simulink model "Buck_BLDC_2023a_4_FaultModel"  (R2024a)
settings: Solver=VariableStepAuto  StartTime=0.0  StopTime=35  RelTol=1e-3  EnableMultiTasking=on
model workspace (MAT data in the model file):
  encoderResolution = 2000
  hallOffset = '0.5'
  indexOffset = 850
  polePairs = '4'
settings Model: Creator=feder  LastModifiedBy=feder
settings OptimizationCC: DefaultParameterBehavior=Inlined
settings DebuggingCC: InheritedTsInSrcMsg=none

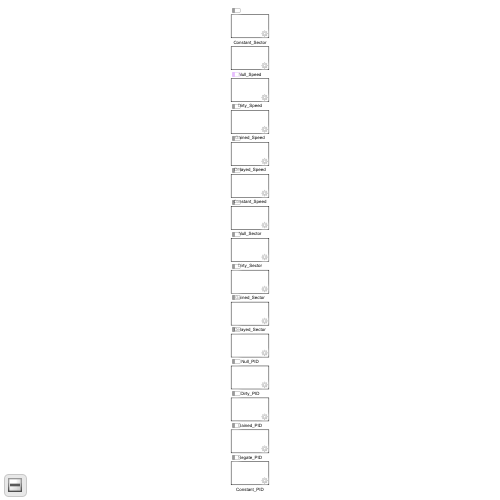
[thumbnail: Simulink's stored preview of the top-level diagram]
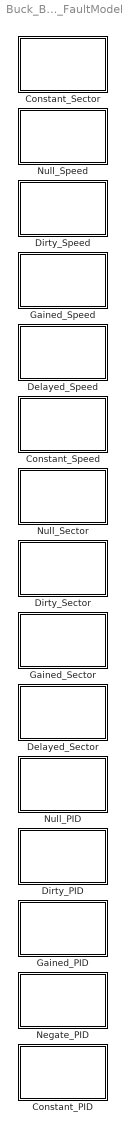
== system Buck_BLDC_2023a_4_FaultModel ==
  Constant_PID : Subsystem  TreatAsAtomicUnit=on  ScheduleAs=Aperiodic partition  PartitionName=PartitionFor_Constant_PID_4698_000977  IsInjectorSS=on
      settings: LibrarySourceBlock=mwfaultlib/Stuck-at-Constant
  Constant_Sector : Subsystem  TreatAsAtomicUnit=on  ScheduleAs=Aperiodic partition  PartitionName=PartitionFor_Constant_Sector_1447_001221  IsInjectorSS=on
      settings: LibrarySourceBlock=mwfaultlib/Stuck-at-Constant
  Constant_Speed : Subsystem  TreatAsAtomicUnit=on  ScheduleAs=Aperiodic partition  PartitionName=PartitionFor_Constant_Speed_1366_012451  IsInjectorSS=on
      settings: LibrarySourceBlock=mwfaultlib/Stuck-at-Constant
  Delayed_Sector : Subsystem  TreatAsAtomicUnit=on  ScheduleAs=Aperiodic partition  PartitionName=PartitionFor_Delayed_Sector_4477_001099  IsInjectorSS=on
      settings: LibrarySourceBlock=mwfaultlib/Unit Delay
  Delayed_Speed : Subsystem  TreatAsAtomicUnit=on  ScheduleAs=Aperiodic partition  PartitionName=PartitionFor_Delayed_Speed_4718_000854  IsInjectorSS=on
      settings: LibrarySourceBlock=mwfaultlib/Unit Delay
  Dirty_PID : Subsystem  TreatAsAtomicUnit=on  ScheduleAs=Aperiodic partition  PartitionName=PartitionFor_Dirty_PID_4657_000854  IsInjectorSS=on
      settings: LibrarySourceBlock=mwfaultlib/Add Noise
  Dirty_Sector : Subsystem  TreatAsAtomicUnit=on  ScheduleAs=Aperiodic partition  PartitionName=PartitionFor_Dirty_Sector_4453_001221  IsInjectorSS=on
      settings: LibrarySourceBlock=mwfaultlib/Add Noise
  Dirty_Speed : Subsystem  TreatAsAtomicUnit=on  ScheduleAs=Aperiodic partition  PartitionName=PartitionFor_Dirty_Speed_7587_001343  IsInjectorSS=on
      settings: LibrarySourceBlock=mwfaultlib/Add Noise
  Gained_PID : Subsystem  TreatAsAtomicUnit=on  ScheduleAs=Aperiodic partition  PartitionName=PartitionFor_Gained_PID_4671_001221  IsInjectorSS=on
      settings: LibrarySourceBlock=mwfaultlib/Gain
  Gained_Sector : Subsystem  TreatAsAtomicUnit=on  ScheduleAs=Aperiodic partition  PartitionName=PartitionFor_Gained_Sector_4467_001099  IsInjectorSS=on
      settings: LibrarySourceBlock=mwfaultlib/Gain
  Gained_Speed : Subsystem  TreatAsAtomicUnit=on  ScheduleAs=Aperiodic partition  PartitionName=PartitionFor_Gained_Speed_4708_000488  IsInjectorSS=on
      settings: LibrarySourceBlock=mwfaultlib/Gain
  Negate_PID : Subsystem  TreatAsAtomicUnit=on  ScheduleAs=Aperiodic partition  PartitionName=PartitionFor_Negate_PID_4687_000854  IsInjectorSS=on
      settings: LibrarySourceBlock=mwfaultlib/Negate Value
  Null_PID : Subsystem  TreatAsAtomicUnit=on  ScheduleAs=Aperiodic partition  PartitionName=PartitionFor_Null_PID_9236_000610  IsInjectorSS=on
      settings: LibrarySourceBlock=mwfaultlib/Stuck-at-Ground
  Null_Sector : Subsystem  TreatAsAtomicUnit=on  ScheduleAs=Aperiodic partition  PartitionName=PartitionFor_Null_Sector_4309_001343  IsInjectorSS=on
      settings: LibrarySourceBlock=mwfaultlib/Stuck-at-Ground
  Null_Speed : Subsystem  TreatAsAtomicUnit=on  IsInjectorSS=on
      settings: LibrarySourceBlock=mwfaultlib/Stuck-at-Ground

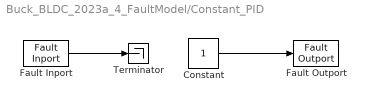
== system Buck_BLDC_2023a_4_FaultModel/Constant_PID ==
  Constant : Constant  SampleTime=-1
  Fault Inport : FaultInport
  Fault Outport : FaultOutport
  Terminator : Terminator
  wires:
  Constant/1 -> Fault Outport/1
  Fault Inport/1 -> Terminator/1

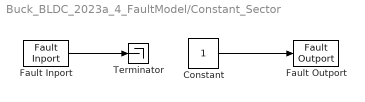
== system Buck_BLDC_2023a_4_FaultModel/Constant_Sector ==
  Constant : Constant  SampleTime=-1
  Fault Inport : FaultInport
  Fault Outport : FaultOutport
  Terminator : Terminator
  wires:
  Constant/1 -> Fault Outport/1
  Fault Inport/1 -> Terminator/1

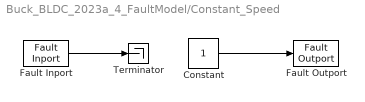
== system Buck_BLDC_2023a_4_FaultModel/Constant_Speed ==
  Constant : Constant  SampleTime=-1
  Fault Inport : FaultInport
  Fault Outport : FaultOutport
  Terminator : Terminator
  wires:
  Constant/1 -> Fault Outport/1
  Fault Inport/1 -> Terminator/1

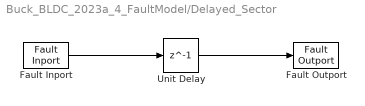
== system Buck_BLDC_2023a_4_FaultModel/Delayed_Sector ==
  Fault Inport : FaultInport
  Fault Outport : FaultOutport
  Unit Delay : Delay  DelayLength=1
  wires:
  Unit Delay/1 -> Fault Outport/1
  Fault Inport/1 -> Unit Delay/1

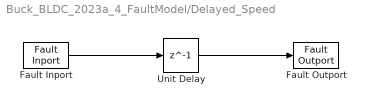
== system Buck_BLDC_2023a_4_FaultModel/Delayed_Speed ==
  Fault Inport : FaultInport
  Fault Outport : FaultOutport
  Unit Delay : Delay  DelayLength=1
  wires:
  Unit Delay/1 -> Fault Outport/1
  Fault Inport/1 -> Unit Delay/1

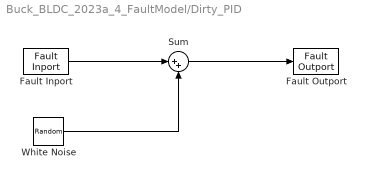
== system Buck_BLDC_2023a_4_FaultModel/Dirty_PID ==
  Fault Inport : FaultInport
  Fault Outport : FaultOutport
  Sum : Sum  Inputs=|++  OutDataTypeStr=Inherit: Inherit via back propagation
  White Noise : RandomNumber  DisableCoverage=on  Seed=[23341]
  wires:
  White Noise/1 -> Sum/2
  Sum/1 -> Fault Outport/1
  Fault Inport/1 -> Sum/1

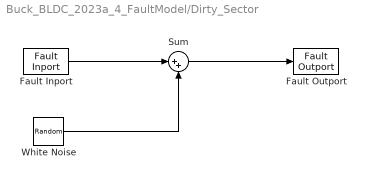
== system Buck_BLDC_2023a_4_FaultModel/Dirty_Sector ==
  Fault Inport : FaultInport
  Fault Outport : FaultOutport
  Sum : Sum  Inputs=|++  OutDataTypeStr=Inherit: Inherit via back propagation
  White Noise : RandomNumber  DisableCoverage=on  Seed=[23341]
  wires:
  White Noise/1 -> Sum/2
  Sum/1 -> Fault Outport/1
  Fault Inport/1 -> Sum/1

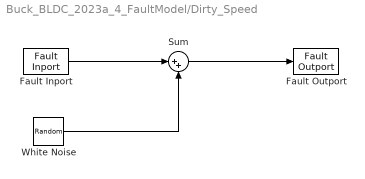
== system Buck_BLDC_2023a_4_FaultModel/Dirty_Speed ==
  Fault Inport : FaultInport
  Fault Outport : FaultOutport
  Sum : Sum  Inputs=|++  OutDataTypeStr=Inherit: Inherit via back propagation
  White Noise : RandomNumber  DisableCoverage=on  Seed=[23341]
  wires:
  White Noise/1 -> Sum/2
  Sum/1 -> Fault Outport/1
  Fault Inport/1 -> Sum/1

== system Buck_BLDC_2023a_4_FaultModel/Gained_PID ==
  Fault Inport : FaultInport
  Fault Outport : FaultOutport
  Gain : Gain  Gain=2  OutDataTypeStr=Inherit: Inherit via back propagation
  wires:
  Gain/1 -> Fault Outport/1
  Fault Inport/1 -> Gain/1

== system Buck_BLDC_2023a_4_FaultModel/Gained_Sector ==
  Fault Inport : FaultInport
  Fault Outport : FaultOutport
  Gain : Gain  Gain=2  OutDataTypeStr=Inherit: Inherit via back propagation
  wires:
  Gain/1 -> Fault Outport/1
  Fault Inport/1 -> Gain/1

== system Buck_BLDC_2023a_4_FaultModel/Gained_Speed ==
  Fault Inport : FaultInport
  Fault Outport : FaultOutport
  Gain : Gain  Gain=2  OutDataTypeStr=Inherit: Inherit via back propagation
  wires:
  Gain/1 -> Fault Outport/1
  Fault Inport/1 -> Gain/1

== system Buck_BLDC_2023a_4_FaultModel/Negate_PID ==
  Fault Inport : FaultInport
  Fault Outport : FaultOutport
  Invert : Gain  Gain=-1
  wires:
  Fault Inport/1 -> Invert/1
  Invert/1 -> Fault Outport/1

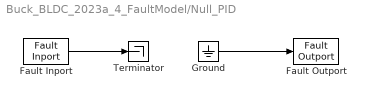
== system Buck_BLDC_2023a_4_FaultModel/Null_PID ==
  Fault Inport : FaultInport
  Fault Outport : FaultOutport
  Ground : Ground
  Terminator : Terminator
  wires:
  Ground/1 -> Fault Outport/1
  Fault Inport/1 -> Terminator/1

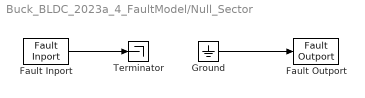
== system Buck_BLDC_2023a_4_FaultModel/Null_Sector ==
  Fault Inport : FaultInport
  Fault Outport : FaultOutport
  Ground : Ground
  Terminator : Terminator
  wires:
  Ground/1 -> Fault Outport/1
  Fault Inport/1 -> Terminator/1

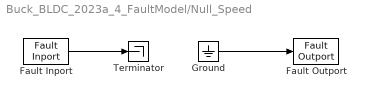
== system Buck_BLDC_2023a_4_FaultModel/Null_Speed ==
  Fault Inport : FaultInport
  Fault Outport : FaultOutport
  Ground : Ground
  Terminator : Terminator
  wires:
  Ground/1 -> Fault Outport/1
  Fault Inport/1 -> Terminator/1
